simulink model "lab2model1"  (R2020a)
settings: Solver=VariableStepAuto  StartTime=0.0  StopTime=20  RelTol=1e-3
settings Model: Creator=Sam  LastModifiedBy=Sam

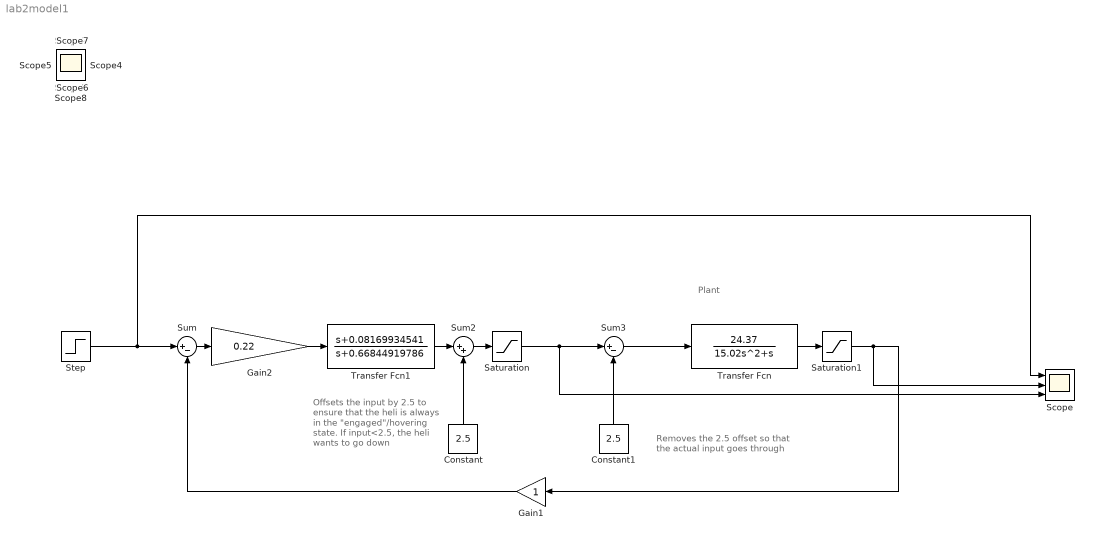
== system lab2model1 ==
  note: Plant
  note: Offsets the input by 2.5 to ensure that the heli is always in the "engaged"/hovering state. If input<2.5, the heli wants to go down
  note: Removes the 2.5 offset so that the actual input goes through
  Constant : Constant  Value=2.5
  Constant1 : Constant  Value=2.5
  Gain1 : Gain
  Gain2 : Gain  Gain=0.22
  Saturation : Saturate  UpperLimit=5  LowerLimit=-5
  Saturation1 : Saturate  UpperLimit=100000  LowerLimit=0
  Scope : Scope  NumInputPorts=3
  Step : Step  After=5  SampleTime=0
  Sum : Sum  Inputs=|+-
  Sum2 : Sum  Inputs=|++
  Sum3 : Sum  Inputs=|+-
  Transfer Fcn : TransferFcn  Numerator=[24.37]  Denominator=[15.02 1 0]
  Transfer Fcn1 : TransferFcn  Numerator=[1 0.08169934541]  Denominator=[1 0.66844919786]
  Scope{1..8} (8 alike) : Scope
  wires:
  Step/1 -> Scope/1, Sum/1
  Sum/1 -> Gain2/1
  Sum2/1 -> Saturation/1
  Saturation/1 -> Scope/3, Sum3/1
  Transfer Fcn/1 -> Saturation1/1
  Gain1/1 -> Sum/2
  Saturation1/1 -> Scope/2, Gain1/1
  Constant/1 -> Sum2/2
  Constant1/1 -> Sum3/2
  Sum3/1 -> Transfer Fcn/1
  Gain2/1 -> Transfer Fcn1/1
  Transfer Fcn1/1 -> Sum2/1
